simulink model "command_processing_test"  (R2016b)
settings: Solver=VariableStepAuto  StartTime=0.0  StopTime=100  RelTol=1e-3
undefined symbols (not defined in the file or in its folder): fsw_params
libraries: simulink x1, command_processing x1
settings Model: Creator=taylorreynolds  LastModifiedBy=taylorreynolds

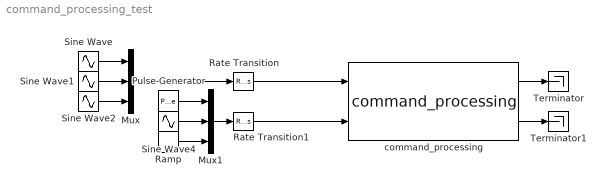
== system command_processing_test ==
  Mux : Mux  Inputs=3
  Mux1 : Mux  Inputs=3
  Pulse Generator : DiscretePulseGenerator  PulseType=Time based  Amplitude=0.15  Period=10  PulseWidth=5
  Ramp : simulink/Sources/Ramp  slope=0.0015  start=0  X0=0
  Rate Transition : RateTransition  OutPortSampleTime=fsw_params.sample_time_s
  Rate Transition1 : RateTransition  OutPortSampleTime=fsw_params.sample_time_s
  Sine Wave : Sin  Amplitude=1e-3  SampleTime=fsw_params.sample_time_s
  Sine Wave1 : Sin  Amplitude=1e-3  Frequency=2  SampleTime=fsw_params.sample_time_s
  Sine Wave2 : Sin  Amplitude=0.5e-4  Phase=-3.14  SampleTime=fsw_params.sample_time_s
  Sine Wave4 : Sin  Amplitude=0.15  SampleTime=fsw_params.sample_time_s
  Terminator : Terminator
  Terminator1 : Terminator
  command_processing : command_processing/command_processing
  wires:
  Sine Wave/1 -> Mux/1
  Sine Wave1/1 -> Mux/2
  Sine Wave2/1 -> Mux/3
  Pulse Generator/1 -> Mux1/1
  Sine Wave4/1 -> Mux1/2
  Ramp/1 -> Mux1/3
  Mux1/1 -> Rate Transition1/1
  command_processing/1 -> Terminator/1
  command_processing/2 -> Terminator1/1
  Rate Transition/1 -> command_processing/1
  Rate Transition1/1 -> command_processing/2
  Mux/1 -> Rate Transition/1
